simulink model "suspension_system"  (R2020a)
settings: Solver=VariableStepAuto  StartTime=0.0  StopTime=10.0  RelTol=1e-3
values from neighbouring files (symbols this model uses):
  b = 50    [command_window.mat]
  k1 = 60    [command_window.mat]
  k2 = 30    [command_window.mat]
  M1 = 0.01    [command_window.mat]
  M2 = 0.1    [command_window.mat]
settings Model: Creator=kolep  LastModifiedBy=kolep

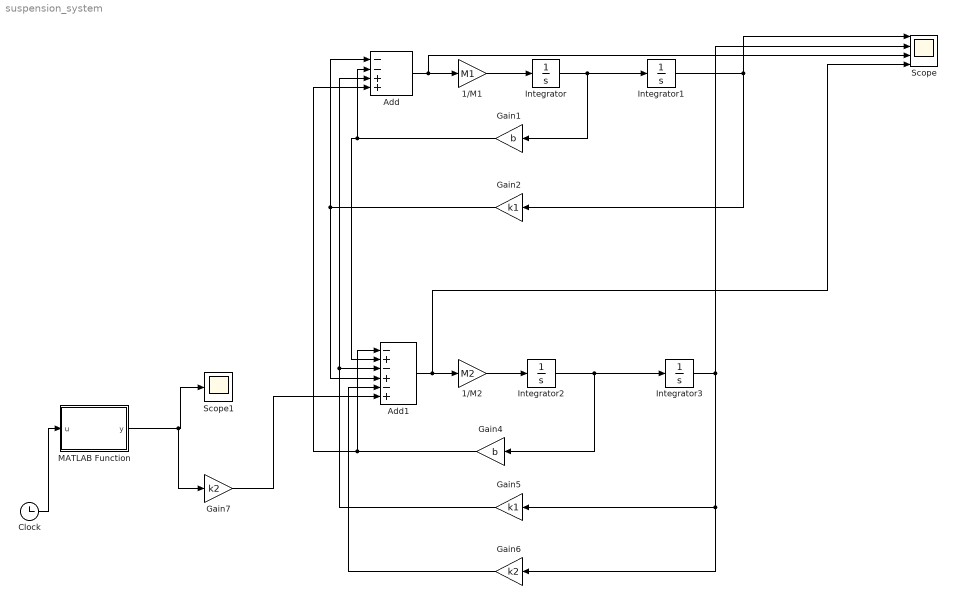
== system suspension_system ==
  1/M1 : Gain  Gain=M1
  1/M2 : Gain  Gain=M2
  Add : Sum  Inputs=--++
  Add1 : Sum  Inputs=-+-+-+
  Clock : Clock
  Gain1 : Gain  Gain=b
  Gain2 : Gain  Gain=k1
  Gain4 : Gain  Gain=b
  Gain5 : Gain  Gain=k1
  Gain6 : Gain  Gain=k2
  Gain7 : Gain  Gain=k2
  Integrator{,1..3} (4 alike) : Integrator
  MATLAB Function : MATLAB Function  TreatAsAtomicUnit=on
  Scope : Scope  NumInputPorts=4
  Scope1 : Scope
  wires:
  Integrator/1 -> Integrator1/1, Gain1/1
  Gain1/1 -> Add1/2, Add/2
  Integrator1/1 -> Gain2/1, Scope/1
  Gain2/1 -> Add1/4, Add/1
  Integrator2/1 -> Integrator3/1, Gain4/1
  Gain4/1 -> Add1/1, Add/4
  Integrator3/1 -> Scope/2, Gain6/1, Gain5/1
  Gain5/1 -> Add/3, Add1/3
  Gain6/1 -> Add1/5
  MATLAB Function/1(y) -> Gain7/1, Scope1/1
  Clock/1 -> MATLAB Function/1(u)
  Add/1 -> Scope/3, 1/M1/1
  1/M1/1 -> Integrator/1
  Add1/1 -> Scope/4, 1/M2/1
  1/M2/1 -> Integrator2/1
  Gain7/1 -> Add1/6

== matlab function suspension_system/MATLAB Function ==
  data: u input; y output
function y = fcn(u)
if ((u >= 0) && (u < 2))
    y = 1;
elseif ((u >= 2) && (u < 5))
    y = sin(2*pi*u);
elseif ((u >= 5) && (u < 8))
    y = 3.5 ;
else
    y = 2;
end
